simulink model "rectifierwith_giveninputformat"  (R2016a)
settings: Solver=FixedStepDiscrete  SolverMode=SingleTasking  StartTime=0.0  StopTime=0.1  FixedStep=1e-07  RelTol=1e-3
undefined symbols (not defined in the file): Acid, Lead
libraries: powerlib x15, electricdrivelib x1
settings Model: Creator=ayaz  LastModifiedBy=Mustafa
settings DataIOCC: ReturnWorkspaceOutputs=on
settings DebuggingCC: SFUnexpectedBacktrackingDiag=error  SFNoUnconditionalDefaultTransitionDiag=error
settings SFSimCC: SimUseLocalCustomCode=on
settings RTWCC: RTWUseLocalCustomCode=on
settings GRTTargetCC: TargetLangStandard=C99 (ISO)  GeneratePreprocessorConditionals=Use local settings
settings ConfigComp: CovMetricSettings=dwe  CovSaveCumulativeToWorkspaceVar=off  CovSaveSingleToWorkspaceVar=off  CovExternalEMLEnable=on

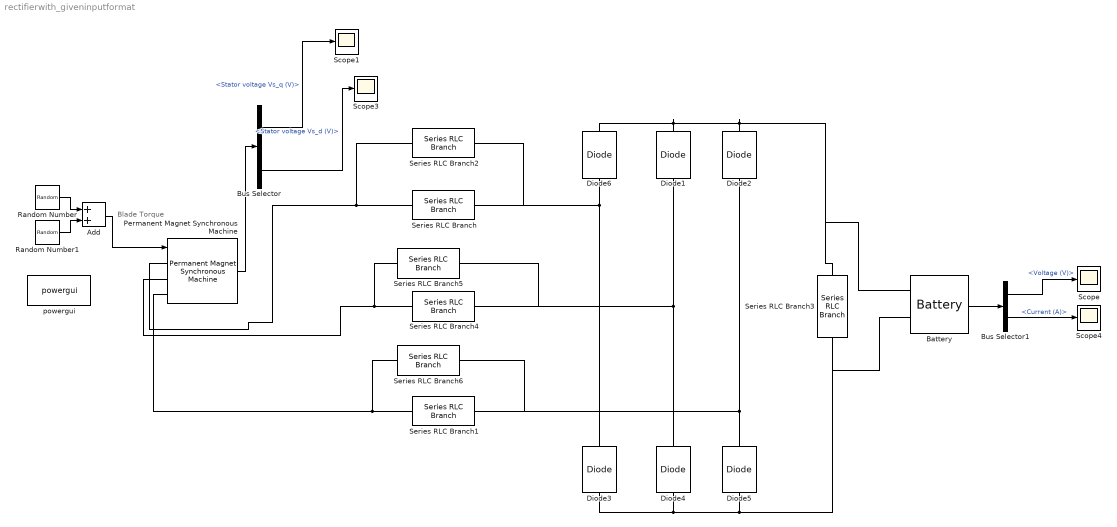
== system rectifierwith_giveninputformat ==
  note: Blade Torque
  Add : Sum
  Battery : electricdrivelib/Extra Sources/Battery  BatType=Lead-Acid  ShowTempParam=off  ThermalPreset=no  NomV=24  NomQ=5.4  SOC=50  Batt_Tr=30  PresetModel=on  MaxQ=5.625  MinV=18  FullV=26.1316  Dis_rate=1.08  R=0.044444  Normal_OP=1.6755  expZone="[24.4342        0.018]"  current=[6.5 13 32.5]  Units=Time  Tci=20  NomT=20  T2=-30  MaxQ2=4.8  FullV2=7.1  Normal_OP2=5.655  expZone2="[6.58           1]"  Rca=0.6  ti=2000  Dp=0
  Bus Selector : BusSelector  OutputSignals=Stator voltage Vs_q (V),Stator voltage Vs_d (V)
  Bus Selector1 : BusSelector  OutputSignals=Voltage (V),Current (A)
  Diode{1..6} (6 alike) : powerlib/Power Electronics/Diode  Ron=0.001  Lon=0  Vf=0.8  IC=0  UseSnubber=off  Rs=500  Cs=250e-9  Measurements=off
  Permanent Magnet Synchronous Machine : powerlib/Machines/Permanent Magnet Synchronous Machine  NbPhases=3  FluxDistribution=Sinusoidal  RotorType=Round  MechanicalLoad=Torque Tm  PresetModel=No  ShowDetailedParameters=on  MeasurementBus=off  Resistance=10.58  Inductance=8.5e-3  dqInductances=[8.5e-3,8.5e-3]  La=0.0167  MachineConstant=Voltage Constant (V_peak L-L / krpm)  Flux=0.60646  VoltageCst=110  TorqueCst=0.90969  Flat=120  Mechanical=[0.00027 0.005024 1 0]  PolePairs=4  InitialConditions=[300,0, 0,0]  InitialConditions5ph=[0 0 0 0 0 0]  TsPowergui=0  TsBlock=-1  RefAngle=90 degrees behind phase A axis (modified Park)
  Random Number : RandomNumber  Mean=-1.6  Variance=0.05  SampleTime=1
  Random Number1 : RandomNumber  Variance=0.1  SampleTime=1e-3
  Scope{,1,3..4} (4 alike) : Scope
  Series RLC Branch : powerlib/Elements/Series RLC Branch  LConnTagsString=__new0  RConnTagsString=__new0  BranchType=L  Resistance=1  Inductance=1e-4  SetiL0=off  InitialCurrent=0  Capacitance=1e-6  Setx0=off  InitialVoltage=0  Measurements=None
  Series RLC Branch1 : powerlib/Elements/Series RLC Branch  LConnTagsString=__new0  RConnTagsString=__new0  BranchType=L  Resistance=1  Inductance=1e-4  SetiL0=off  InitialCurrent=0  Capacitance=1e-6  Setx0=off  InitialVoltage=0  Measurements=None
  Series RLC Branch2 : powerlib/Elements/Series RLC Branch  LConnTagsString=__new0  RConnTagsString=__new0  BranchType=R  Resistance=1e12  Inductance=1e-3  SetiL0=off  InitialCurrent=0  Capacitance=1e-6  Setx0=off  InitialVoltage=0  Measurements=None
  Series RLC Branch3 : powerlib/Elements/Series RLC Branch  LConnTagsString=__new0  RConnTagsString=__new0  BranchType=C  Resistance=1  Inductance=1e-3  SetiL0=off  InitialCurrent=0  Capacitance=1e-9  Setx0=off  InitialVoltage=0  Measurements=None
  Series RLC Branch4 : powerlib/Elements/Series RLC Branch  LConnTagsString=__new0  RConnTagsString=__new0  BranchType=L  Resistance=1  Inductance=1e-4  SetiL0=off  InitialCurrent=0  Capacitance=1e-6  Setx0=off  InitialVoltage=0  Measurements=None
  Series RLC Branch5 : powerlib/Elements/Series RLC Branch  LConnTagsString=__new0  RConnTagsString=__new0  BranchType=R  Resistance=1e12  Inductance=1e-3  SetiL0=off  InitialCurrent=0  Capacitance=1e-6  Setx0=off  InitialVoltage=0  Measurements=None
  Series RLC Branch6 : powerlib/Elements/Series RLC Branch  LConnTagsString=__new0  RConnTagsString=__new0  BranchType=R  Resistance=1e12  Inductance=1e-3  SetiL0=off  InitialCurrent=0  Capacitance=1e-6  Setx0=off  InitialVoltage=0  Measurements=None
  powergui : powerlib/powergui  Priority=1  SimulationMode=Discrete  SolverType=Tustin/Backward Euler (TBE)  SampleTime=1e-7  frequency=60  SPID=on  DisableSnubberDevices=off  DisableRonSwitches=off  DisableVfSwitches=off  SwTol=0  DisplayEquations=off  Interpol=off  ExternalGateDelay=off  methode=off  Ts=100  FunctionMessages=off  echomessages=off  HookPort=off  EnableUseOfTLC=off  x0status=blocks  frequencyindice=0  Pbase=100e6  ErrMax=1e-4  Iterations=50  UnitsV=kV  UnitsW=MW  buscounter=0  RestoreLinks=warning  ResistiveCurrentMeasurement=off  Frange=[0:2:500]  Ylog=off  Xlog=on  ShowGrid=off  save=off  variable=ZData  structure=0  ZoomFFT=off  StartTime=0.0  cycles=1  DisplayStyle=1  fundamental=60  FreqAxis=off  MaxFrequency=1000  frequencyindicesteady=1  RmsSteady=1  display=off
  wires:
  Random Number/1 -> Add/1
  Random Number1/1 -> Add/2
  Add/1 -> Permanent Magnet Synchronous Machine/1
  Battery/1 -> Bus Selector1/1
  Permanent Magnet Synchronous Machine/1 -> Bus Selector/1
  Bus Selector/1 -> Scope1/1  "<Stator voltage Vs_q (V)>"
  Bus Selector/2 -> Scope3/1  "<Stator voltage Vs_d (V)>"
  Bus Selector1/1 -> Scope/1  "<Voltage (V)>"
  Bus Selector1/2 -> Scope4/1  "<Current (A)>"
  connections:
  Series RLC Branch/LConn1 -- Series RLC Branch2/LConn1 -- Permanent Magnet Synchronous Machine/LConn1
  Series RLC Branch4/LConn1 -- Series RLC Branch5/LConn1 -- Permanent Magnet Synchronous Machine/LConn2
  Series RLC Branch1/LConn1 -- Series RLC Branch6/LConn1 -- Permanent Magnet Synchronous Machine/LConn3
  Diode2/LConn1 -- Series RLC Branch6/RConn1 -- Series RLC Branch1/RConn1 -- Diode5/RConn1
  Diode1/LConn1 -- Series RLC Branch5/RConn1 -- Series RLC Branch4/RConn1 -- Diode4/RConn1
  Diode6/LConn1 -- Series RLC Branch2/RConn1 -- Series RLC Branch/RConn1 -- Diode3/RConn1
  Diode1/RConn1 -- Diode6/RConn1 -- Battery/LConn1 -- Series RLC Branch3/LConn1 -- Diode2/RConn1
  Diode5/LConn1 -- Series RLC Branch3/RConn1 -- Battery/LConn2 -- Diode3/LConn1 -- Diode4/LConn1
